simulink model "DiagramaDeBloques"  (R2023b)
settings: Solver=VariableStepAuto  StartTime=0.0  StopTime=10.0  RelTol=1e-3
InitFcn:
  | %% Parámetros del Geófono (Base para el diseño)
  | % Conservamos los parámetros mecánicos necesarios para la desintonización
  | fn  = 10;                % Frecuencia natural del geófono (Hz)
  | wn  = 2*pi*fn;           % Frecuencia natural (rad/s)
  | h0  = 0.25;              % Amortiguamiento intrínseco del geófono
  | 
  | %% 1. Amplificador de Entrada (INA)
  | % Modelado como un filtro pasa bajas de primer polo (ideal).
  | ganancia_INA = 100;      % Ganancia V/V deseada
  | fc_INA = 5e6;          % Frecuencia de corte del INA (Hz) - Ajustable
  | wc_INA = 2*pi*fc_INA;
  | 
  | % TF = ganancia_INA * ( wc_INA / (s + wc_INA) )
  | Amplificador_n = [ganancia_INA * wc_INA];
  | Amplificador_d = [1, wc_INA];
  | 
  | %% 2. Filtro BandPass (Acondicionamiento / Desintonización)
  | % Diseñado en base a la dinámica del compensador ideal
  | fLow = 0.1;
  | wLow = 2*pi*fLow;
  | h1   = wn/(2*wLow);      % Nuevo factor de amortiguamiento (zeta del compensador)
  | 
  | % Numerador: 2*(h1-h0)*wn*s
  | BandPass_n = [2*(h1-h0)*wn, 0];
  | % Denominador: s^2 + 2*h1*wn*s + wn^2
  | BandPass_d = [1, 2*h1*wn, wn^2];
  | 
  | %% 3. Filtro LowPass (Antialias)
  | % Filtro de segundo orden parametrizable ideal
  | f0_lp   = 120;           % Frecuencia de corte del filtro antialias (Hz)
  | w0_lp   = 2*pi*f0_lp;    % Frecuencia natural (rad/s)
  | zeta_lp = 0.707;         % Factor de amortiguamiento (Ej: 0.707 para Butterworth ideal)
  | 
  | % TF = w0^2 / (s^2 + 2*zeta*w0*s + w0^2)
  | Antialias_n = [w0_lp^2];
  | Antialias_d = [1, 2*zeta_lp*w0_lp, w0_lp^2];
  | 
  | %% 4. Ganancia y ADC Delta-Sigma
  | PGA_gain = 3/4;          % Ganancia de entrada previa al ADC
  | Fs = 1000;             % Frecuencia de muestreo del ADC (Ej: 256 kHz)
  | Fs_adc = Fs*64;
  | Ts = 1/Fs;               % Tiempo de muestreo del ADC
  | Ts_adc = 1/Fs_adc;
  | %% 5. Filtro FIR Digital (firls)
  | % Parámetros de la etapa de decimación
  | orden_fir = 64;          % Orden del filtro (ajustable)
  | 
  | % Frecuencias para firls (normalizadas respecto a Fs/2 de la etapa correspondiente)
  | % Asumiendo diseño para la primera etapa digital (antes de decimar):
  | f_pass_norm = 0.1;       % Frecuencia de fin de banda de paso (normalizada 0 a 1)
  | f_stop_norm = 0.2;       % Frecuencia de inicio de banda de rechazo (normalizada)
  | 
  | % Vector de frecuencias [0, f_pass, f_stop, 1]
  | F_fir = [0, f_pass_norm, f_stop_norm, 1];
  | 
  | % Amplitudes deseadas en cada banda [1 a 1 (pass), 0 a 0 (stop)]
  | A_fir =;
  | 
  | % Pesos (ponderación) para las bandas: [Peso_PassBand, Peso_StopBand]
  | % Ponderar más la banda de rechazo ayuda a mejorar la atenuación del ruido de cuantización
  | W_fir =;
  | 
  | % Generación de coeficientes con firls
  | FIR_filter = firls(orden_fir, F_fir, A_fir, W_fir);
undefined symbols (not defined in the file or in its folder): Hbpd, Hbpn, Hd_d, Hd_n, Hfa, Hg_ad, Hg_an, K_u
libraries: dspmlti4 x3
settings Model: Creator=elias  LastModifiedBy=elias

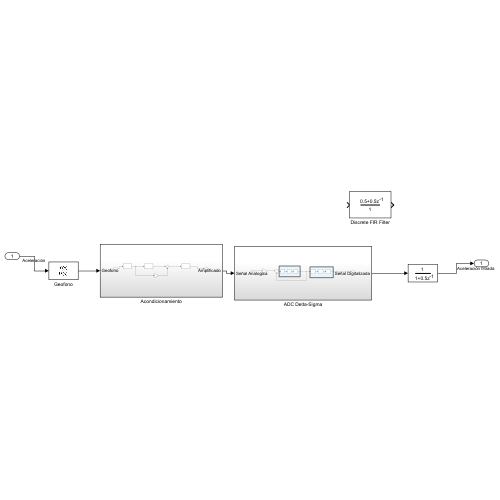
[thumbnail: Simulink's stored preview of the top-level diagram]
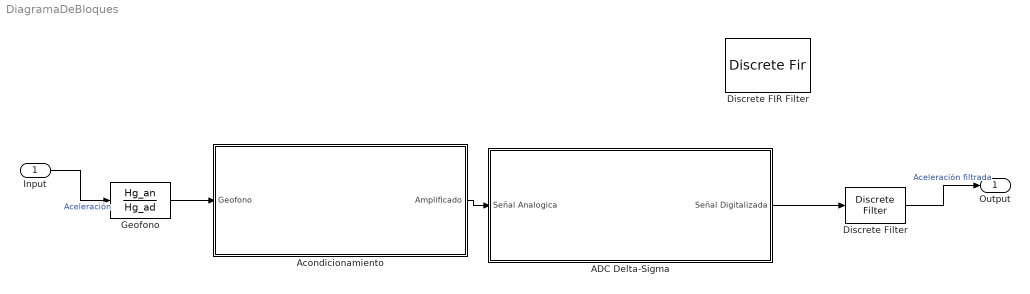
== system DiagramaDeBloques ==
  Input : Inport
  ADC Delta-Sigma : Subsystem
  Acondicionamiento : Subsystem
  Discrete FIR Filter : DiscreteFir
  Discrete Filter : DiscreteFilter
  Geofono : TransferFcn  Numerator=Hg_an  Denominator=Hg_ad
  Output : Outport
  wires:
  Input/1 -> Geofono/1  "Aceleración"
  Geofono/1 -> Acondicionamiento/1(Geofono)
  Acondicionamiento/1(Amplificado) -> ADC Delta-Sigma/1(Señal Analogica)
  ADC Delta-Sigma/1(Señal Digitalizada) -> Discrete Filter/1
  Discrete Filter/1 -> Output/1  "Aceleración filtrada"

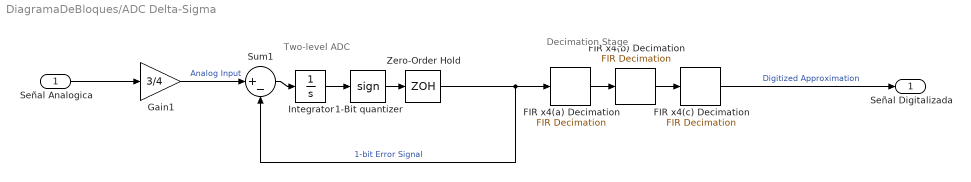
== system DiagramaDeBloques/ADC Delta-Sigma ==
  note: Two-level ADC
  note: Decimation Stage
  Señal Analogica : Inport
  1-Bit quantizer : Signum
  FIR x4(a) Decimation : dspmlti4/FIR Decimation  FilterSource=Dialog parameters  h=fir1(31,0.15)  D=4  filtStruct=Direct form  FilterObject=Hm_firdecim  framing=Allow multirate processing  AllowArbitraryInputLength=off  inputOffset=0  outputBufInitCond=0  roundingMode=Floor  overflowMode=off  firstCoeffDataTypeStr=Inherit: Same word length as input  firstCoeffMin=[]  firstCoeffMax=[]  firstCoeffLastDataTypeStr=Inherit: Same word length as input  accumDataTypeStr=Inherit: Same as product output  accumLastDataTypeStr=Inherit: Same as product output  outputMin=[]  outputMax=[]
  FIR x4(b) Decimation : dspmlti4/FIR Decimation  FilterSource=Dialog parameters  h=fir1(31,0.15)  D=4  filtStruct=Direct form  FilterObject=Hm_firdecim  framing=Allow multirate processing  AllowArbitraryInputLength=off  inputOffset=0  outputBufInitCond=0  roundingMode=Floor  overflowMode=off  firstCoeffDataTypeStr=Inherit: Same word length as input  firstCoeffMin=[]  firstCoeffMax=[]  firstCoeffLastDataTypeStr=Inherit: Same word length as input  accumDataTypeStr=Inherit: Same as product output  accumLastDataTypeStr=Inherit: Same as product output  outputMin=[]  outputMax=[]
  FIR x4(c) Decimation : dspmlti4/FIR Decimation  FilterSource=Dialog parameters  h=fir1(31,0.15)  D=4  filtStruct=Direct form  FilterObject=Hm_firdecim  framing=Allow multirate processing  AllowArbitraryInputLength=off  inputOffset=0  outputBufInitCond=0  roundingMode=Floor  overflowMode=off  firstCoeffDataTypeStr=Inherit: Same word length as input  firstCoeffMin=[]  firstCoeffMax=[]  firstCoeffLastDataTypeStr=Inherit: Same word length as input  accumDataTypeStr=Inherit: Same as product output  accumLastDataTypeStr=Inherit: Same as product output  outputMin=[]  outputMax=[]
  Gain1 : Gain  Gain=3/4  SaturateOnIntegerOverflow=on  OutDataTypeStr=Inherit: Same as input  ParamDataTypeStr=Inherit: Same as input
  Integrator : Integrator
  Sum1 : Sum  Inputs=|+-  InputSameDT=on  SaturateOnIntegerOverflow=on  OutDataTypeStr=Inherit: Same as first input
  Zero-Order Hold : ZeroOrderHold  SampleTime=1/512E3
  Señal Digitalizada : Outport
  wires:
  Integrator/1 -> 1-Bit quantizer/1
  Zero-Order Hold/1 -> FIR x4(a) Decimation/1, Sum1/2  "1-bit Error Signal"
  FIR x4(b) Decimation/1 -> FIR x4(c) Decimation/1
  FIR x4(a) Decimation/1 -> FIR x4(b) Decimation/1
  Sum1/1 -> Integrator/1
  1-Bit quantizer/1 -> Zero-Order Hold/1
  Señal Analogica/1 -> Gain1/1
  Gain1/1 -> Sum1/1  "Analog Input"
  FIR x4(c) Decimation/1 -> Señal Digitalizada/1  "Digitized Approximation"

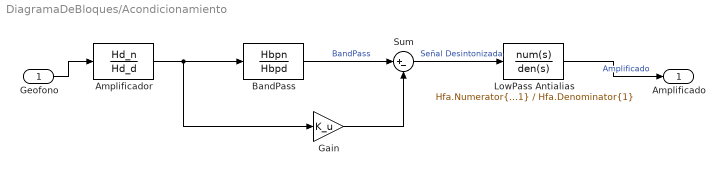
== system DiagramaDeBloques/Acondicionamiento ==
  Geofono : Inport
  Amplificador : TransferFcn  Numerator=Hd_n  Denominator=Hd_d
  BandPass : TransferFcn  Numerator=Hbpn  Denominator=Hbpd
  Gain : Gain  Gain=K_u
  LowPass Antialias : TransferFcn  Numerator=Hfa.Numerator{1}  Denominator=Hfa.Denominator{1}
  Sum : Sum  Inputs=|+-
  Amplificado : Outport
  wires:
  Amplificador/1 -> BandPass/1, Gain/1
  LowPass Antialias/1 -> Amplificado/1  "Amplificado"
  Geofono/1 -> Amplificador/1
  Sum/1 -> LowPass Antialias/1  "Señal Desintonizada"
  Gain/1 -> Sum/2
  BandPass/1 -> Sum/1  "BandPass"
